simulink model "s360159_sim"  (R2025b)
settings: Solver=VariableStepAuto  StartTime=0.0  StopTime=t_sim  RelTol=1e-3
values from neighbouring files (symbols this model uses):
  delta_d2 = 0    [s360159_design.m]
  delta_r = 0.5    [s360159_design.m]
  Ts = 10e-3    (= 0.01)    [s360159_design.m]    (also in s360159_design_MPC.m = 0.05)
libraries: cstblocks x2
settings Model: Creator=giovannimasi  LastModifiedBy=giovannimasi

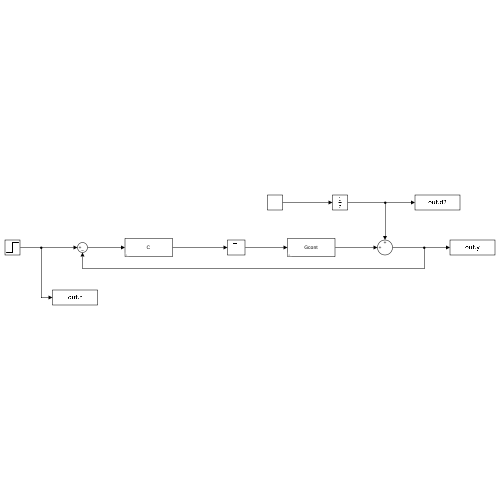
[thumbnail: Simulink's stored preview of the top-level diagram]
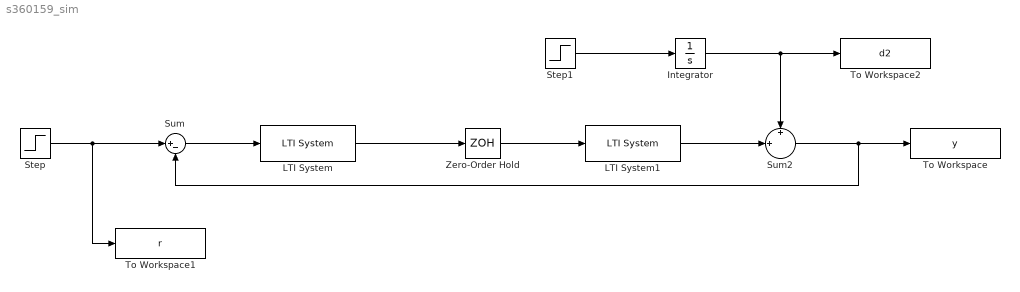
== system s360159_sim ==
  Integrator : Integrator
  LTI System : cstblocks/LTI System  sys=C  IC=[]  PadeOrder=0
  LTI System1 : cstblocks/LTI System  sys=Gcont  IC=[]  PadeOrder=0
  Step : Step  Time=0  After=delta_r  SampleTime=Ts
  Step1 : Step  Time=0  After=delta_d2  SampleTime=Ts
  Sum : Sum  Inputs=|+-
  Sum2 : Sum  Inputs=+|+||
  To Workspace : ToWorkspace  VariableName=y  SaveFormat=Timeseries  SampleTime=Ts
  To Workspace1 : ToWorkspace  VariableName=r  SaveFormat=Timeseries  SampleTime=Ts
  To Workspace2 : ToWorkspace  VariableName=d2  SaveFormat=Timeseries  SampleTime=Ts
  Zero-Order Hold : ZeroOrderHold  SampleTime=Ts
  wires:
  Step/1 -> To Workspace1/1, Sum/1
  Sum/1 -> LTI System/1
  LTI System/1 -> Zero-Order Hold/1
  Zero-Order Hold/1 -> LTI System1/1
  LTI System1/1 -> Sum2/2
  Sum2/1 -> To Workspace/1, Sum/2
  Step1/1 -> Integrator/1
  Integrator/1 -> To Workspace2/1, Sum2/1
